simulink model "taha_project_trail1"  (R2025b)
settings: Solver=VariableStepAuto  StartTime=0.0  StopTime=0.4  RelTol=1e-3
libraries: spsSeriesRLCBranchLib x4, spsMosfetLib x1, dspstat3 x1, spsPVArrayLib x1, rllib x1, simulink x1, spsVoltageMeasurementLib x1, spsDiodeLib x1, sps_lib x1
settings Model: SimulationMode=accelerator  Creator=DELL  LastModifiedBy=DELL

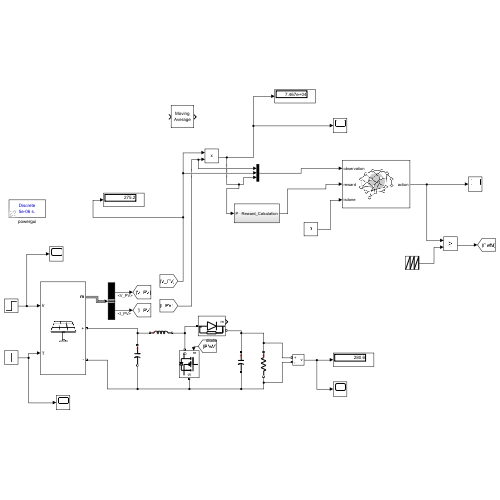
[thumbnail: Simulink's stored preview of the top-level diagram]
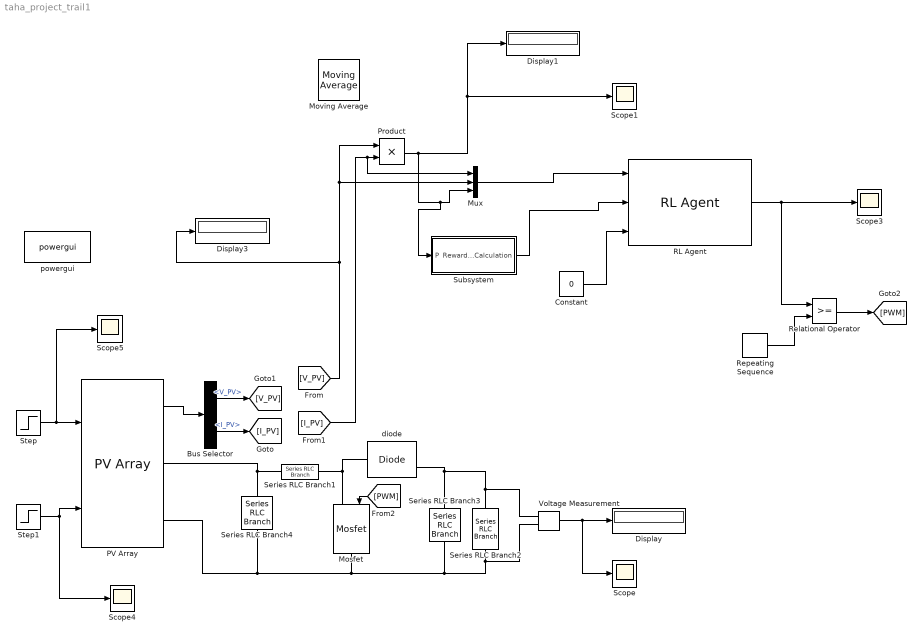
== system taha_project_trail1 ==
  Bus Selector : BusSelector  OutputSignals=V_PV,I_PV
  Constant : Constant  Value=0
  Display : Display
  Display1 : Display
  Display3 : Display
  Mosfet : spsMosfetLib/Mosfet  Ron=0.1  Lon=0  Rd=0.01  Vfd=0  IC=0  Rs=1e5  Cs=inf  Measurements=off
  Moving Average : dspstat3/Moving Average  Method=Sliding window  ForgettingFactorPort=off  SpecifyWindowLength=on  WindowLength=200  OverlapLength=199  AllowArbitraryInputLength=off  ForgettingFactor=0.9  SimulateUsing=Interpreted execution
  Mux : Mux  Inputs=3
  PV Array : spsPVArrayLib/PV Array  Npar=47  Nser=10  PlotType=array @ 25 deg.C & specified irradiances  S_vec=[ 500]  Temp_C_vec="[ 45 25  ]"  ModuleName=Solartech Energy ASC-6P-54-215  PlotWhenSelected=off  Pm=215.0162  Ncell=54  Voc=33.44  Isc=8.52  Vm=26.81  Im=8.02  beta_Voc_pc=-0.36  alpha_Isc_pc=0.06  beta_Voc=-0.12038  alpha_Isc=0.005112  IL=8.5504  I0=2.8918e-10  nI=1.0002  Rsh=356.7155  Rs=0.32117  RobustModel=off  RobustCellTemperature=313.3991  BAL=on  Tc=1e-6  Tfilter=5e-5
  Product : Product
  RL Agent : rllib/RL Agent  Agent=agent  ExternalActionAsInput=off  ProvideLastAction=off  ProvideCumRwd=off  TreatAsDirectFeedthrough=on  UseStrictObservationDataTypes=off
  Relational Operator : RelationalOperator  OutDataTypeStr=boolean  RndMeth=Simplest  InputSameDT=off
  Repeating Sequence : simulink/Sources/Repeating Sequence  rep_seq_t=[0 0.0002]  rep_seq_y=[0 1]
  Scope{,1,3..5} (5 alike) : Scope
      Scope settings: ActiveDisplayYMinimum=-1407.5687924126476  ActiveDisplayYMaximum=1351.0105498140549
      Scope1 settings: ActiveDisplayYMinimum=-53588.9044666789  ActiveDisplayYMaximum=126813.34534423858
      Scope3 settings: ActiveDisplayYMinimum=-0.0045352836877667188  ActiveDisplayYMaximum=0.0094626790134126563  DataLoggingVariableName=ScopeData3
      Scope4 settings: ActiveDisplayYMinimum=12.703767055261455  ActiveDisplayYMaximum=51.110842887068927  DataLoggingVariableName=ScopeData4
      Scope5 settings: ActiveDisplayYMinimum=325  ActiveDisplayYMaximum=1075  DataLoggingVariableName=ScopeData5
  Series RLC Branch1 : spsSeriesRLCBranchLib/Series RLC Branch  LConnTagsString=__new0  RConnTagsString=__new0  BranchType=L  Resistance=1  Inductance=1.6e-3  SetiL0=off  InitialCurrent=0  Capacitance=1e-6  Setx0=off  InitialVoltage=0  Measurements=None
  Series RLC Branch2 : spsSeriesRLCBranchLib/Series RLC Branch  LConnTagsString=__new0  RConnTagsString=__new0  BranchType=R  Resistance=1.06  Inductance=1e-3  SetiL0=off  InitialCurrent=0  Capacitance=1e-6  Setx0=off  InitialVoltage=0  Measurements=None
  Series RLC Branch3 : spsSeriesRLCBranchLib/Series RLC Branch  LConnTagsString=__new0  RConnTagsString=__new0  BranchType=C  Resistance=0.0001  Inductance=1e-3  SetiL0=off  InitialCurrent=0  Capacitance=3300e-6  Setx0=off  InitialVoltage=0  Measurements=None
  Series RLC Branch4 : spsSeriesRLCBranchLib/Series RLC Branch  LConnTagsString=__new0  RConnTagsString=__new0  BranchType=C  Resistance=0.0001  Inductance=1e-3  SetiL0=off  InitialCurrent=0  Capacitance=3300e-6  Setx0=off  InitialVoltage=0  Measurements=None
  Step : Step  Time=0.025  Before=400  After=1000  SampleTime=0
  Step1 : Step  Time=0.025  Before=15  After=45  SampleTime=0
  Subsystem : Subsystem
  Voltage Measurement : spsVoltageMeasurementLib/Voltage Measurement  PhasorSimulation=off  OutputType=Complex  PSBequivalent=0
  diode : spsDiodeLib/Diode  Ron=0.001  Lon=0  Vf=0.8  IC=0  UseSnubber=0  Rs=500  Cs=250e-9  Measurements=on
  powergui : sps_lib/powergui  Priority=1  SimulationMode=Discrete  SampleTime=5e-6  frequency=60  Iterations=50  frequencyindice=0  Pbase=100e6  ErrMax=1e-4  UnitsV=kV  UnitsW=MW  buscounter=0  FunctionMessages=off  echomessages=off  EnableUseOfTLC=off  CurrentSourceSwitches=off  DisableSnubberDevices=off  DisableRonSwitches=off  DisableVfSwitches=off  DisplayEquations=off  AutomaticDiscreteSolvers=off  SolverType=Tustin/Backward Euler (TBE)  Interpol=off  ExternalGateDelay=off  methode=off  Ts=100  x0status=blocks  SPID=on  SwTol=0  HookPort=off  NonlinearTolerance=1e-4  nMaxIteration=100  ContinueOnMaxIteration=off  RestoreLinks=warning  ResistiveCurrentMeasurement=off  Frange=[0:2:500]  Ylog=off  Xlog=on  ShowGrid=off  save=off  variable=ZData  structure=0  ZoomFFT=off  StartTime=0.0  cycles=1  DisplayStyle=1  fundamental=60  FreqAxis=off  MaxFrequency=1000  frequencyindicesteady=1  RmsSteady=1  display=off
  wires:
  Bus Selector/2 -> [I_PV]  "<I_PV>"
  Step1/1 -> Scope4/1, PV Array/2
  Bus Selector/1 -> [V_PV]  "<V_PV>"
  Voltage Measurement/1 -> Scope/1, Display/1
  [PWM] -> Mosfet/1
  PV Array/1 -> Bus Selector/1
  [V_PV] -> Mux/2, Product/1, Display3/1
  [I_PV] -> Mux/1, Product/2
  Repeating Sequence/1 -> Relational Operator/2
  Relational Operator/1 -> [PWM]
  Product/1 -> Subsystem/1(P), Mux/3, Display1/1, Scope1/1
  RL Agent/1 -> Scope3/1, Relational Operator/1
  Mux/1 -> RL Agent/1
  Constant/1 -> RL Agent/3
  Subsystem/1(Reward_Calculation) -> RL Agent/2
  Step/1 -> Scope5/1, PV Array/1
  connections:
  PV Array/RConn2 -- Voltage Measurement/LConn2 -- Series RLC Branch2/RConn1 -- Series RLC Branch3/RConn1 -- Mosfet/RConn1 -- Series RLC Branch4/RConn1
  Series RLC Branch3/LConn1 -- Series RLC Branch2/LConn1 -- Voltage Measurement/LConn1 -- diode/RConn1
  Series RLC Branch1/RConn1 -- Mosfet/LConn1 -- diode/LConn1
  Series RLC Branch1/LConn1 -- PV Array/RConn1 -- Series RLC Branch4/LConn1

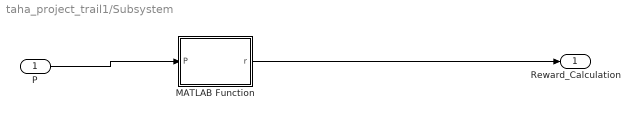
== system taha_project_trail1/Subsystem ==
  P : Inport
  MATLAB Function : MATLAB Function  TreatAsAtomicUnit=on
  Reward_Calculation : Outport
  wires:
  P/1 -> MATLAB Function/1(P)
  MATLAB Function/1(r) -> Reward_Calculation/1

== matlab function taha_project_trail1/Subsystem/MATLAB Function ==
  data: P input; r output
function r = f(P)
    persistent P_prev;
    if isempty(P_prev); P_prev = 0; end
    
    delta_P = P - P_prev;
    
    % DEAD ZONE: Ignore noise smaller than 50 Watts
    if delta_P > 50      
        r = 20;          % Real Power Increase
    elseif delta_P < -50 
        r = -60;         % Real Power Drop
    else                
        % Steady state: Reward high absolute power
        r = P * 0.001; 
    end
    
    P_prev = P;
end
